simulink library "golayLib"  (R2014b)
settings: Solver=ode45  StartTime=0.0  StopTime=10.0  RelTol=1e-3
undefined symbols (not defined in the file): D_128, W_128
settings Model: Creator=cyarp  LastModifiedBy=cyarp

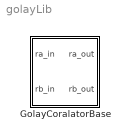
== system golayLib ==
  GolayCoralatorBase : Subsystem  mask(Golay Correlator Base){dSub=D_128(1), wSub=W_128(1)}
      mask prompts: dSub "D Parameter"; wSub "W Parameter"
      mask help: Base Unit of a Golay Correlator

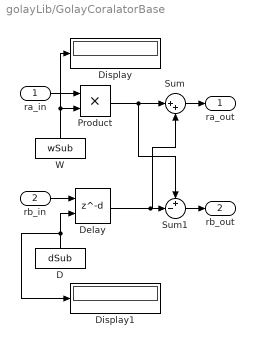
== system golayLib/GolayCoralatorBase ==
  ra_in : Inport  OutDataTypeStr=int16
  rb_in : Inport  Port=2  OutDataTypeStr=int16
  D : Constant  Value=dSub  OutDataTypeStr=Inherit: Inherit via back propagation
  Delay : Delay  DelayLengthSource=Input port  DelayLength=dSub  DelayLengthUpperLimit=1000  InitialCondition=0  DiagnosticForOutOfRangeDelayLength=Error  UseCircularBuffer=on
      settings: InputPortMap=u0,p1
  Display : Display
  Display1 : Display
  Product : Product
  Sum : Sum  Inputs=|++
  Sum1 : Sum  Inputs=+-|
  W : Constant  Value=wSub  OutDataTypeStr=Inherit: Inherit via back propagation
  ra_out : Outport  OutDataTypeStr=int16
  rb_out : Outport  Port=2  OutDataTypeStr=int16
  wires:
  Sum/1 -> ra_out/1
  Sum1/1 -> rb_out/1
  ra_in/1 -> Product/1
  W/1 -> Product/2, Display/1
  rb_in/1 -> Delay/1
  D/1 -> Display1/1, Delay/2
  Delay/1 -> Sum/2, Sum1/2
  Product/1 -> Sum1/1, Sum/1
